simulink model "Problema8_2_Preditor_Teste"  (R2018b)
settings: Solver=VariableStepAuto  StartTime=0.0  StopTime=25  RelTol=1e-3
values from neighbouring files (symbols this model uses):
  A = [ -3 0; 1 0 ]    [Problema8_2.m]
  B = [ 1; 0]    [Problema8_2.m]
  C = [ 0 1 ]    [Problema8_2.m]
  Ca = [1 0;0 1]    [Problema8_2.m]
  D = 0    [Problema8_2.m]
  Da = [0;0]    [Problema8_2.m]
  h = 0.2    [Problema8_2.m]
  L = [0 1] * inv(Wc) * (phi^2 + p1 * phi + p2 * eye(2))    [Problema8_2.m]
  Lc = ganho_dc/( C * inv(eye(2) - phi_cl ) * gama )    [Problema8_2.m]
  x0 = [ 0 0 ]'    [Problema8_2.m]
settings Model: Creator=Asus  LastModifiedBy=fredericovaz
settings SFSimCC: SimUseLocalCustomCode=off
settings RTWCC: RTWUseLocalCustomCode=off
settings CodeAppCC: StateflowObjectComments=on

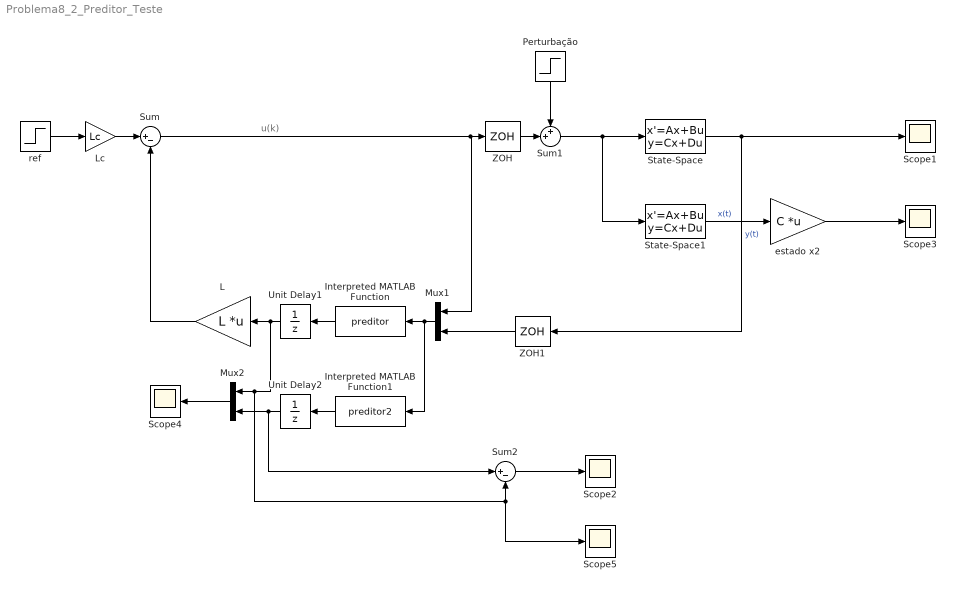
== system Problema8_2_Preditor_Teste ==
  note: u(k)
  Interpreted MATLAB Function : MATLABFcn  MATLABFcn=preditor  OutputDimensions=2
  Interpreted MATLAB Function1 : MATLABFcn  MATLABFcn=preditor2  OutputDimensions=2
  L : Gain  Gain=L  Multiplication=Matrix(K*u) (u vector)
  Lc : Gain  Gain=Lc
  Mux1 : Mux  Inputs=2
  Mux2 : Mux  Inputs=2
  Perturbação : Step  Time=15  After=0.3  SampleTime=0
  Scope{1..5} (5 alike) : Scope
  State-Space : StateSpace  A=A  B=B  C=C  D=D  InitialCondition=x0
  State-Space1 : StateSpace  A=A  B=B  C=Ca  D=Da  InitialCondition=x0
  Sum : Sum  Inputs=|+-
  Sum1 : Sum  Inputs=++|
  Sum2 : Sum  Inputs=|+-
  Unit Delay1 : UnitDelay  SampleTime=-1
  Unit Delay2 : UnitDelay  SampleTime=-1
  ZOH : ZeroOrderHold  SampleTime=h
  ZOH1 : ZeroOrderHold  SampleTime=h
  "estado x2 " : Gain  Gain=C  Multiplication=Matrix(K*u) (u vector)
  "ref " : Step  Time=5  After=0.4  SampleTime=0
  wires:
  ZOH/1 -> Sum1/2
  L/1 -> Sum/2
  Sum1/1 -> State-Space1/1, State-Space/1
  Lc/1 -> Sum/1
  "ref "/1 -> Lc/1
  Sum/1 -> Mux1/1, ZOH/1
  Perturbação/1 -> Sum1/1
  State-Space1/1 -> "estado x2 "/1  "x(t)"
  Mux1/1 -> Interpreted MATLAB Function1/1, Interpreted MATLAB Function/1
  Interpreted MATLAB Function/1 -> Unit Delay1/1
  Unit Delay1/1 -> Mux2/1, Scope5/1, Sum2/2, L/1
  ZOH1/1 -> Mux1/2
  State-Space/1 -> ZOH1/1, Scope1/1  "y(t)"
  "estado x2 "/1 -> Scope3/1
  Interpreted MATLAB Function1/1 -> Unit Delay2/1
  Unit Delay2/1 -> Sum2/1, Mux2/2
  Mux2/1 -> Scope4/1
  Sum2/1 -> Scope2/1
